simulink model "testmodel"  (R2022b)
settings: Solver=VariableStepAuto  StartTime=0.0  StopTime=1000  RelTol=1e-3
libraries: simulink x3
settings Model: Creator=86134  LastModifiedBy=86134

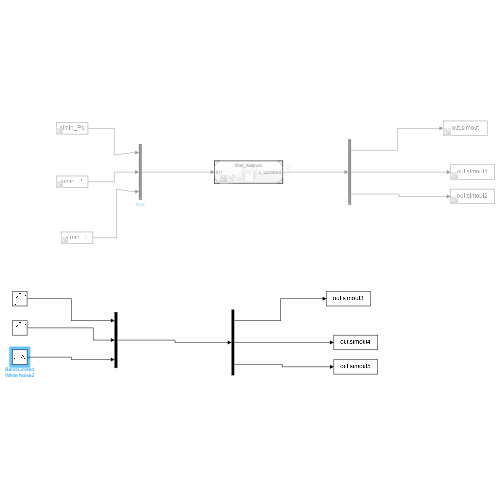
[thumbnail: Simulink's stored preview of the top-level diagram]
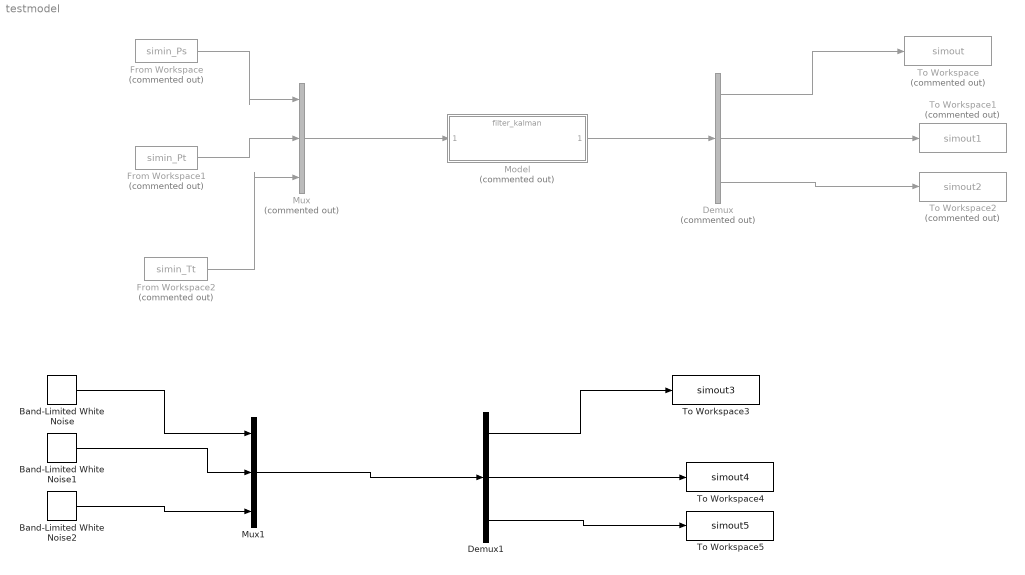
== system testmodel ==
  Band-Limited White Noise : simulink/Sources/Band-Limited White Noise  Cov=[0.04]  Ts=0.1  seed=[23341]
  Band-Limited White Noise1 : simulink/Sources/Band-Limited White Noise  Cov=[0.02]  Ts=0.1  seed=[23341]
  Band-Limited White Noise2 : simulink/Sources/Band-Limited White Noise  Cov=[0.03]  Ts=0.1  seed=[23341]
  Demux : Demux  Commented=on  Outputs=3
  Demux1 : Demux  Outputs=3
  From Workspace : FromWorkspace  Commented=on  VariableName=simin_Ps
  From Workspace1 : FromWorkspace  Commented=on  VariableName=simin_Pt
  From Workspace2 : FromWorkspace  Commented=on  VariableName=simin_Tt
  Model : ModelReference  Commented=on  ModelNameDialog=filter_kalman.slx  SimulationMode=Normal  ModelReferenceVersion=1.38
  Mux : Mux  Commented=on  Inputs=3
  Mux1 : Mux  Inputs=3
  To Workspace : ToWorkspace  Commented=on  VariableName=simout  SaveFormat=Timeseries  SampleTime=-1
  To Workspace1 : ToWorkspace  Commented=on  VariableName=simout1  SaveFormat=Timeseries  SampleTime=-1
  To Workspace2 : ToWorkspace  Commented=on  VariableName=simout2  SaveFormat=Timeseries  SampleTime=-1
  To Workspace3 : ToWorkspace  VariableName=simout3  SaveFormat=Timeseries  SampleTime=-1
  To Workspace4 : ToWorkspace  VariableName=simout4  SaveFormat=Timeseries  SampleTime=-1
  To Workspace5 : ToWorkspace  VariableName=simout5  SaveFormat=Timeseries  SampleTime=-1
  wires:
  From Workspace/1 -> Mux/1
  From Workspace1/1 -> Mux/2
  From Workspace2/1 -> Mux/3
  Model/1 -> Demux/1
  Mux/1 -> Model/1
  Demux/1 -> To Workspace/1
  Demux/2 -> To Workspace1/1
  Demux/3 -> To Workspace2/1
  Mux1/1 -> Demux1/1
  Demux1/3 -> To Workspace5/1
  Demux1/1 -> To Workspace3/1
  Demux1/2 -> To Workspace4/1
  Band-Limited White Noise/1 -> Mux1/1
  Band-Limited White Noise1/1 -> Mux1/2
  Band-Limited White Noise2/1 -> Mux1/3
